simulink model "comparator"  (R2023b)
settings: Solver=VariableStepAuto  StartTime=0.0  StopTime=10.0  RelTol=1e-3
settings Model: Creator=1234  LastModifiedBy=1234

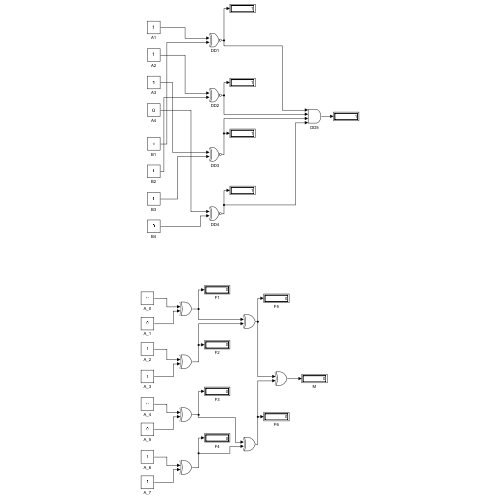
[thumbnail: Simulink's stored preview of the top-level diagram]
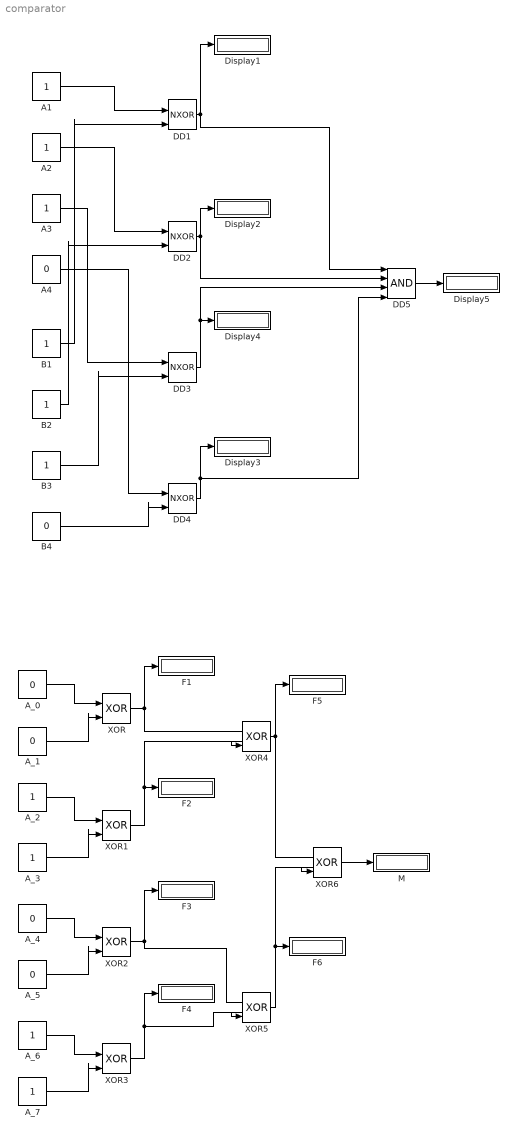
== system comparator ==
  A1 : Constant
  A2 : Constant
  A3 : Constant
  A4 : Constant  Value=0
  A_{0..1,4..5} (4 alike) : Constant  Value=0
  A_{2..3,6..7} (4 alike) : Constant
  B1 : Constant
  B2 : Constant
  B3 : Constant
  B4 : Constant  Value=0
  DD{1..4} (4 alike) : Logic  Operator=NXOR  IconShape=distinctive  AllPortsSameDT=off  OutDataTypeStr=boolean
  DD5 : Logic  Inputs=4  IconShape=distinctive  AllPortsSameDT=off  OutDataTypeStr=boolean
  Display{1..5} (5 alike) : Display
  F{1..6} (6 alike) : Display
  M : Display
  XOR{,1..6} (7 alike) : Logic  Operator=XOR  IconShape=distinctive  AllPortsSameDT=off  OutDataTypeStr=boolean
  wires:
  A1/1 -> DD1/1
  A2/1 -> DD2/1
  A3/1 -> DD3/1
  A4/1 -> DD4/1
  B1/1 -> DD1/2
  B2/1 -> DD2/2
  B3/1 -> DD3/2
  B4/1 -> DD4/2
  DD1/1 -> Display1/1, DD5/1
  DD2/1 -> Display2/1, DD5/2
  DD3/1 -> DD5/3, Display4/1
  DD4/1 -> DD5/4, Display3/1
  DD5/1 -> Display5/1
  A_0/1 -> XOR/1
  A_1/1 -> XOR/2
  A_3/1 -> XOR1/2
  A_2/1 -> XOR1/1
  A_6/1 -> XOR3/1
  A_7/1 -> XOR3/2
  A_5/1 -> XOR2/2
  A_4/1 -> XOR2/1
  XOR/1 -> XOR4/1, F1/1
  XOR1/1 -> XOR4/2, F2/1
  XOR2/1 -> XOR5/1, F3/1
  XOR3/1 -> F4/1, XOR5/2
  XOR5/1 -> F6/1, XOR6/2
  XOR4/1 -> F5/1, XOR6/1
  XOR6/1 -> M/1
